simulink model "Ejercicio1"  (R2025a)
settings: Solver=ode8  StartTime=0.0  StopTime=10  FixedStep=0.01  RelTol=1e-3
values from neighbouring files (symbols this model uses):
  G_array = cat(3, G_cell{:})    [Constantes1.m]    (also in Constantes2.m)
  K_array = cat(3, K_cell{:})    [Constantes1.m]    (also in Constantes2.m)
  P_array = cat(3, P_cell{:})    [Constantes1.m]    (also in Constantes2.m)
settings Model: Creator=440G5  LastModifiedBy=440G5

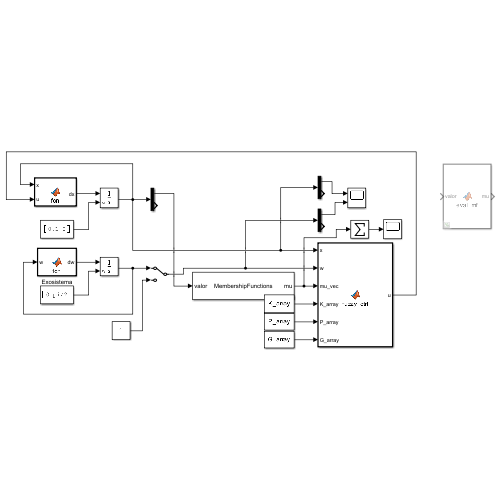
[thumbnail: Simulink's stored preview of the top-level diagram]
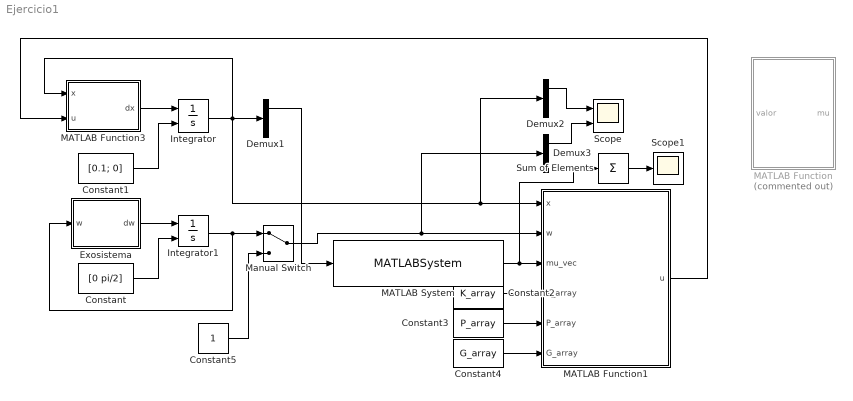
== system Ejercicio1 ==
  Constant : Constant  Value=[0 pi/2]
  Constant1 : Constant  Value=[0.1; 0]
  Constant2 : Constant  Value=K_array
  Constant3 : Constant  Value=P_array
  Constant4 : Constant  Value=G_array
  Constant5 : Constant
  Demux1 : Demux  Outputs=2
  Demux2 : Demux  Outputs=2
  Demux3 : Demux  Outputs=2
  Exosistema : MATLAB Function  TreatAsAtomicUnit=on
  Integrator : Integrator  InitialConditionSource=external
  Integrator1 : Integrator  InitialConditionSource=external
  MATLAB Function : MATLAB Function  Commented=on  TreatAsAtomicUnit=on
  MATLAB Function1 : MATLAB Function  TreatAsAtomicUnit=on
  MATLAB Function3 : MATLAB Function  TreatAsAtomicUnit=on
  MATLAB System : MATLABSystem  System=MembershipFunctions  N=5  Range=[ -15, 15 ]  InputIsRadians=true  SimulateUsing=Interpreted execution
      mask Type: MembershipFunctions
  Manual Switch : ManualSwitch
  Scope : Scope  NumInputPorts=2
      settings: ActiveDisplayYMinimum=-1.7975318202039194  ActiveDisplayYMaximum=1.3616000836433615
  Scope1 : Scope
      settings: ActiveDisplayYMinimum=0.99999999999989564  ActiveDisplayYMaximum=1.0000000000001141
  Sum of Elements : Sum  Inputs=+
  wires:
  MATLAB System/1 -> Sum of Elements/1, MATLAB Function1/3(mu_vec)
  Integrator/1 -> Demux1/1, MATLAB Function1/1(x), Demux2/1, MATLAB Function3/1(x)
  MATLAB Function3/1(dx) -> Integrator/1
  Constant1/1 -> Integrator/2
  Exosistema/1(dw) -> Integrator1/1
  Constant/1 -> Integrator1/2
  Integrator1/1 -> Manual Switch/1, Exosistema/1(w)
  Demux2/1 -> Scope/1
  Demux1/1 -> MATLAB System/1
  Constant2/1 -> MATLAB Function1/4(K_array)
  Constant3/1 -> MATLAB Function1/5(P_array)
  Constant4/1 -> MATLAB Function1/6(G_array)
  Sum of Elements/1 -> Scope1/1
  MATLAB Function1/1(u) -> MATLAB Function3/2(u)
  Demux3/1 -> Scope/2
  Manual Switch/1 -> Demux3/1, MATLAB Function1/2(w)
  Constant5/1 -> Manual Switch/2

== matlab function Ejercicio1/MATLAB Function1 ==
  data: x input; u output; w input; mu_vec input; K_array input; P_array input; G_array input
function u = fuzzy_ctrl(x, w, mu_vec, K_array, P_array, G_array)
% Control difuso generalizado con N reglas

    N = length(mu_vec);
    u_num = 0;
    u_den = 0;

    for i = 1:N
        Ki = K_array(:,:,i);
        Pi = P_array(:,:,i);
        Gi = G_array(:,:,i);

        ui = -Ki*x + (Gi - Ki*Pi)*w;

        u_num = u_num + mu_vec(i)*ui;
        u_den = u_den + mu_vec(i);
    end

    if u_den > 0
        u = u_num / u_den;
    else
        u = 0;
    end
end

== matlab function Ejercicio1/MATLAB Function ==
  data: mu output; valor input
function mu = eval_mf(valor)
% Número de funciones de membresía (constante)
N = 5;
rango = [-15 15];

% Inicializar salida con tamaño fijo
mu = zeros(1,N);

rmin = rango(1);
rmax = rango(2);
step = (rmax - rmin) / (N - 1);
centers = rmin:step:rmax;

for i = 1:N
    if i == 1
        if valor <= centers(1)
            mu(i) = 1;
        elseif valor >= centers(2)
            mu(i) = 0;
        else
            mu(i) = (centers(2) - valor) / (centers(2) - centers(1));
        end

    elseif i == N
        if valor >= centers(end)
            mu(i) = 1;
        elseif valor <= centers(end-1)
            mu(i) = 0;
        else
            mu(i) = (valor - centers(end-1)) / (centers(end) - centers(end-1));
        end

    else
        left = centers(i-1);
        mid  = centers(i);
        right = centers(i+1);

        if valor == mid
            mu(i) = 1;
        elseif valor > left && valor < mid
            mu(i) = (valor - left) / (mid - left);
        elseif valor > mid && valor < right
            mu(i) = (right - valor) / (right - mid);
        else
            mu(i) = 0;
        end
    end
end

== matlab function Ejercicio1/Exosistema ==
  data: w input; dw output
function dw = fcn(w)

dw = [0 10; -10 0]*w;

== matlab function Ejercicio1/MATLAB Function3 ==
  data: x input; u input; dx output
function dx  = fcn(x, u)
g = 9.81;  
l = 1;     
m = 1;     
b = 0.5;   

x1 = x(1);  
x2 = x(2);

dx1 = x2;
dx2 = (g/l)*sin(x1) - (b/(m*l^2))*x2 + u/(m*l^2);

dx = [dx1; dx2];

y = x1;
